simulink model "driver_controller"  (R2017a)
settings: Solver=VariableStepAuto  StartTime=0.0  StopTime=10.0  RelTol=1e-3
undefined symbols (not defined in the file): D, I, P
settings Model: Creator=devon  LastModifiedBy=devon

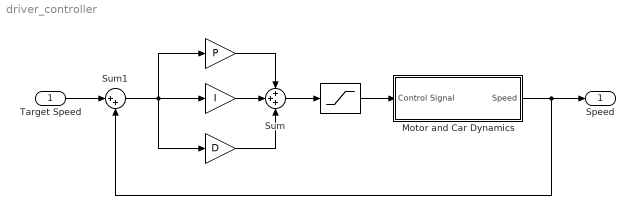
== system driver_controller ==
  Target Speed : Inport
  " " : Gain  Gain=P
  "  " : Gain  Gain=I
  "   " : Gain  Gain=D
  "    " : Saturate  UpperLimit=1  LowerLimit=-1
  Motor and Car Dynamics : Subsystem
  Sum : Sum  Inputs=+++
  Sum1 : Sum  Inputs=|++
  Speed : Outport
  wires:
  Sum1/1 -> "   "/1, " "/1, "  "/1
  " "/1 -> Sum/1
  "  "/1 -> Sum/2
  "   "/1 -> Sum/3
  Sum/1 -> "    "/1
  "    "/1 -> Motor and Car Dynamics/1(Control Signal)
  Motor and Car Dynamics/1(Speed) -> Sum1/2, Speed/1
  Target Speed/1 -> Sum1/1

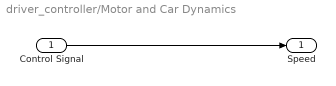
== system driver_controller/Motor and Car Dynamics ==
  Control Signal : Inport
  Speed : Outport
  wires:
  Control Signal/1 -> Speed/1
